simulink model "proyecto"  (R2021a)
settings: Solver=VariableStepAuto  StartTime=0.0  StopTime=50  RelTol=1e-3
undefined symbols (not defined in the file or in its folder): kp5_0, Ti5_0
libraries: cstblocks x1
settings Model: Creator=OKM  LastModifiedBy=gabri

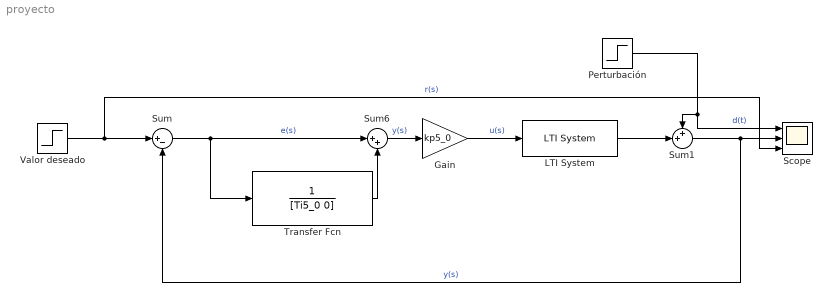
== system proyecto ==
  Gain : Gain  Gain=kp5_0
  LTI System : cstblocks/LTI System  sys=P_0  IC=[]
  Perturbación : Step  Time=20  After=10  SampleTime=0
  Scope : Scope  NumInputPorts=3
  Sum : Sum  Inputs=|+-
  Sum1 : Sum  Inputs=++|
  Sum6 : Sum  Inputs=|++
  Transfer Fcn : TransferFcn  Denominator=[Ti5_0 0]
  Valor deseado : Step  Time=0  After=80  SampleTime=0
  wires:
  Valor deseado/1 -> Scope/3, Sum/1  "r(s)"
  Sum1/1 -> Scope/2, Sum/2  "y(s)"
  Perturbación/1 -> Scope/1, Sum1/1  "d(t)"
  Sum6/1 -> Gain/1  "y(s)"
  Sum/1 -> Sum6/1, Transfer Fcn/1  "e(s)"
  LTI System/1 -> Sum1/2
  Transfer Fcn/1 -> Sum6/2
  Gain/1 -> LTI System/1  "u(s)"
